simulink model "ej7"  (Simulink 7.0)
settings: Solver=ode45  StartTime=0.0  StopTime=10  RelTol=1e-3
settings Model: Creator=alumno  LastModifiedBy=alumno

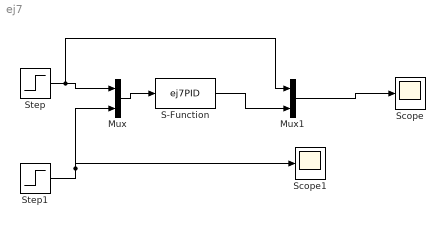
== system ej7 ==
  Mux : Mux  Inputs=2
  Mux1 : Mux  Inputs=2
  S-Function : S-Function  FunctionName=ej7PID  Parameters=1 .1 10 10 0.01
  Scope : Scope
  Scope1 : Scope
  Step : Step  SampleTime=0
  Step1 : Step  Time=2  SampleTime=0
  wires:
  Mux/1 -> S-Function/1
  Step/1 -> Mux/1, Mux1/1
  Mux1/1 -> Scope/1
  S-Function/1 -> Mux1/2
  Step1/1 -> Mux/2, Scope1/1
